simulink library "state_estimation"  (R2016b)
settings: Solver=VariableStepAuto  StartTime=0.0  StopTime=10.0  RelTol=1e-3
libraries: extended_kalman_filter_lib x1, triad_coarse_estimator x1
settings Model: Creator=sexymathemagician  LastModifiedBy=sexymathemagician

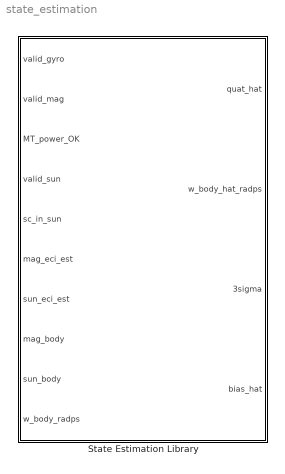
== system state_estimation ==
  State Estimation Library : Subsystem

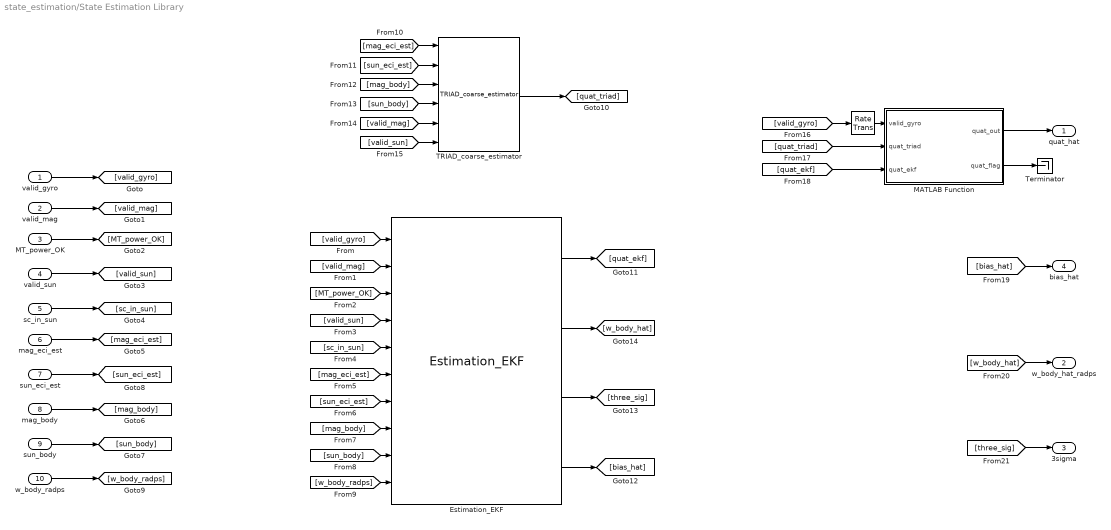
== system state_estimation/State Estimation Library ==
  valid_gyro : Inport
  valid_mag : Inport  Port=2
  MT_power_OK : Inport  Port=3
  "valid_sun " : Inport  Port=4
  sc_in_sun : Inport  Port=5
  mag_eci_est : Inport  Port=6
  sun_eci_est : Inport  Port=7
  mag_body : Inport  Port=8
  sun_body : Inport  Port=9
  w_body_radps : Inport  Port=10
  " " : RateTransition  X0=fsw_params.estimation.ic.rt_valid_gyro  OutPortSampleTime=fsw_params.estimation.sample_time_s
  "Estimation_EKF " : extended_kalman_filter_lib/Estimation_EKF 
  MATLAB Function : MATLAB Function  TreatAsAtomicUnit=on
  TRIAD_coarse_estimator : triad_coarse_estimator/TRIAD_coarse_estimator
  Terminator : Terminator
  quat_hat : Outport
  w_body_hat_radps : Outport  Port=2
  3sigma : Outport  Port=3
  bias_hat : Outport  Port=4
  wires:
  valid_gyro/1 -> [valid_gyro]
  valid_mag/1 -> [valid_mag]
  "valid_sun "/1 -> [valid_sun]
  mag_body/1 -> [mag_body]
  sun_body/1 -> [sun_body]
  MT_power_OK/1 -> [MT_power_OK]
  [bias_hat] -> bias_hat/1
  [three_sig] -> 3sigma/1
  [w_body_hat] -> w_body_hat_radps/1
  MATLAB Function/1(quat_out) -> quat_hat/1
  sc_in_sun/1 -> [sc_in_sun]
  mag_eci_est/1 -> [mag_eci_est]
  sun_eci_est/1 -> [sun_eci_est]
  [valid_gyro] -> "Estimation_EKF "/1
  [valid_mag] -> "Estimation_EKF "/2
  [MT_power_OK] -> "Estimation_EKF "/3
  [valid_sun] -> "Estimation_EKF "/4
  [sc_in_sun] -> "Estimation_EKF "/5
  [mag_eci_est] -> "Estimation_EKF "/6
  [sun_eci_est] -> "Estimation_EKF "/7
  [mag_body] -> "Estimation_EKF "/8
  [sun_body] -> "Estimation_EKF "/9
  w_body_radps/1 -> [w_body_radps]
  [w_body_radps] -> "Estimation_EKF "/10
  [mag_eci_est] -> TRIAD_coarse_estimator/1
  [sun_eci_est] -> TRIAD_coarse_estimator/2
  [mag_body] -> TRIAD_coarse_estimator/3
  [sun_body] -> TRIAD_coarse_estimator/4
  [valid_mag] -> TRIAD_coarse_estimator/5
  [valid_sun] -> TRIAD_coarse_estimator/6
  TRIAD_coarse_estimator/1 -> [quat_triad]
  "Estimation_EKF "/1 -> [quat_ekf]
  [valid_gyro] -> " "/1
  " "/1 -> MATLAB Function/1(valid_gyro)
  [quat_triad] -> MATLAB Function/2(quat_triad)
  [quat_ekf] -> MATLAB Function/3(quat_ekf)
  "Estimation_EKF "/4 -> [bias_hat]
  "Estimation_EKF "/3 -> [three_sig]
  "Estimation_EKF "/2 -> [w_body_hat]
  MATLAB Function/2(quat_flag) -> Terminator/1

== matlab function state_estimation/State Estimation Library/MATLAB Function ==
  data: valid_gyro input; quat_out output; quat_triad input; quat_ekf input; quat_flag output
function [quat_out, quat_flag] = quat_picker(valid_gyro, quat_triad, quat_ekf)
%#codegen

% logic for selecting the quaternion estimate
% if the gyro is invalid, use the TRIAD quat estimate
% if the EKF has not converged, use the TRIAD quat estimate
% otherwise, use the EKF quat estimate
% 
% the flag is set to 1 if the EKF estimate is chosen, and 2 if TRIAD 
%
% modified: April 27, 2018 by M. Hudoba de Badyn


if valid_gyro == 1 
    % if gyro is valid, check convergence
    
    % CONVERGENCE TEST CODE HERE
    % since the descope, we don't want to switch between TRIAD and EKF
    % midfly. In the future, we may want to switch between TRIAD and EKF if
    % the 3-sigma bounds become too high or something. In the case that is
    % decided, change this converge_flag code to something less trivial.
    converge_flag = 1;
    
    if converge_flag == 1
        quat_out = quat_ekf;
        quat_flag = 1;
    else
        quat_out = quat_triad;
        quat_flag = 2;
    end
else
    quat_out = quat_triad;
    quat_flag = 2;
end


end
